simulink model "test_SHState"  (Simulink 6.5)
settings: Solver=VariableStepDiscrete  StartTime=0.0  StopTime=100  RelTol=1e-3
undefined symbols (not defined in the file or in its folder): sigbuilder_block
libraries: xbsIndex_r4 x7, nort_sysgenlib x1
settings Model: Creator=nort  LastModifiedBy=nort

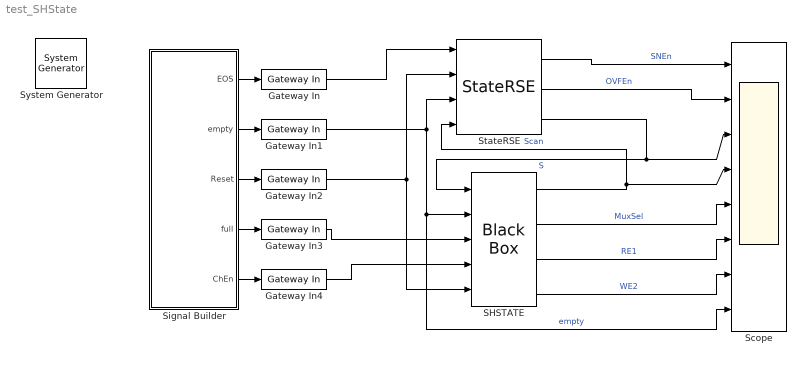
== system test_SHState ==
  " System Generator" : xbsIndex_r4/ System Generator  Tag=genX  SystemSampleTime=-1  xilinxfamily=virtex4  part=xc4vsx35  speed=-10  package=ff668  synthesis_tool=XST  directory=./netlist  testbench=off  simulink_period=1  sysclk_period=10  incr_netlist=off  trim_vbits=Everywhere in SubSystem  dbl_ovrd=According to Block Masks  core_generation=According to Block Masks  run_coregen=off  deprecated_control=off  eval_field=0  block_type=sysgen
      settings: block_version=9.2.01
  Gateway In{,1..3} (4 alike) : xbsIndex_r4/Gateway In  arith_type=Boolean  n_bits=16  bin_pt=14  quantization="Round  (unbiased: +/- Inf)"  overflow=Saturate  period=1  dbl_ovrd=off  timing_constraint=None  locs_specified=off  LOCs={}  block_type=gatewayin
      settings: infoedit="Gateway in block.  Converts inputs of type Simulink integer, double and fixed point to  Xilinx fixed point type.<P><P>Hardware notes:  In hardware these blocks become top level input ports."  block_version=9.2.01
  Gateway In4 : xbsIndex_r4/Gateway In  arith_type=Unsigned  n_bits=3  bin_pt=0  quantization="Round  (unbiased: +/- Inf)"  overflow=Saturate  period=1  dbl_ovrd=off  timing_constraint=None  locs_specified=off  LOCs={}  block_type=gatewayin
      settings: infoedit="Gateway in block.  Converts inputs of type Simulink integer, double and fixed point to  Xilinx fixed point type.<P><P>Hardware notes:  In hardware these blocks become top level input ports."  block_version=9.2.01
  SHSTATE : xbsIndex_r4/Black Box  init_code=SHSTATE_config  sim_method=ISE Simulator  block_type=blackbox2
      settings: infoedit="Incorporates black box HDL and simulation model into a System Generator design.<P><P>You must supply a Black Box with certain information about the HDL component you would like to bring into System Generator. This information is provided through a Matlab function.<P><P>When \"Simulation mode\" is set to \"Inactive\", you will typically want to provide a separate simulation model by using a Simulation Multiplexer.<P>When \"Simulation mode\" is set to \"External co-simulator\", you must include a ModelSim block in the design."  block_version=9.2.01
  Scope : Scope  NumInputPorts=8
      settings: TimeRange=100  YMin=-0.25~-0.25~-0.25~-0.25~-0.1~-0.25~-0.25~-0.25  YMax=1.25~1.25~1.25~1.25~10~1.25~1.25~1.25
  Signal Builder : Subsystem  Tag=STV Subsys  LoadFcn=sigbuilder_block('load');  StartFcn=sigbuilder_block('start');  StopFcn=sigbuilder_block('stop');  ClipboardFcn=sigbuilder_block('clipboard');  mask(Sigbuilder block){}
      mask help: Sigbuilder GUI
      mask init:
      | if ~strcmp(get_param(bdroot(gcbh),'SimulationStatus'),'stopped') tuvar = sigbuilder_block('maskInit'); end
      settings: CopyFcn=sigbuilder_block('copy');  DeleteFcn=sigbuilder_block('delete');  ModelCloseFcn=sigbuilder_block('modelClose');  PreSaveFcn=sigbuilder_block('preSave');  NameChangeFcn=sigbuilder_block('namechange');  OpenFcn=sigbuilder_block('open',[24 64.5 474 399.75 ]);  CloseFcn=sigbuilder_block('close');
      mask Display: plot(0,0,100,100,[10,10,40,40,10],[80,20,20,80,80],[40,10],[50,50], [40,27,10],[65,72,56],[40,25,25,10],[28,28,43,43]);
  StateRSE : nort_sysgenlib/StateRSE  SystemSampleTime=-1
  wires:
  StateRSE/3 -> Scope/3, SHSTATE/1  "S"
  Signal Builder/1(EOS) -> Gateway In/1
  Signal Builder/2(empty) -> Gateway In1/1
  Signal Builder/3(Reset) -> Gateway In2/1
  Signal Builder/4(full) -> Gateway In3/1
  Signal Builder/5(ChEn) -> Gateway In4/1
  StateRSE/1 -> Scope/1  "SNEn"
  StateRSE/2 -> Scope/2  "OVFEn"
  SHSTATE/2 -> Scope/5  "MuxSel"
  SHSTATE/3 -> Scope/6  "RE1"
  SHSTATE/4 -> Scope/7  "WE2"
  Gateway In/1 -> StateRSE/1
  Gateway In1/1 -> StateRSE/3, SHSTATE/2, Scope/8  "empty"
  Gateway In2/1 -> SHSTATE/5, StateRSE/2
  Gateway In3/1 -> SHSTATE/3
  Gateway In4/1 -> SHSTATE/4
  SHSTATE/1 -> Scope/4, StateRSE/4  "Scan"

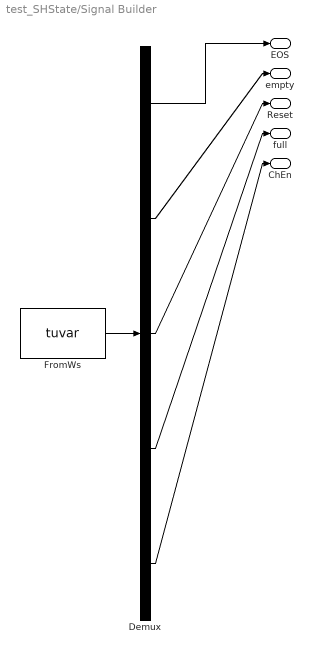
== system test_SHState/Signal Builder ==
  Demux : Demux  Tag=STV Demux  Outputs=5
  FromWs : FromWorkspace  Tag=STV FromWs  VariableName=tuvar  SampleTime=0  SigBuilderData=DataTag1  VnvData=DataTag2
      SigBuilderData=|
      | channels(1).label = 'EOS'
      | channels(1).allXData = {[0 4 6 40 40 41 41 100], [0 4 6 40 40 41 41 100], [0 4 6 40 40 41 41 100], [0 4 6 40 40 41 41 100], [0 4 6 40 40 41 41 100]}
      | channels(1).allYData = {[0 0 0 0 1 1 0 0], [0 0 0 0 1 1 0 0], [0 0 0 0 1 1 0 0], [0 0 0 0 1 1 0 0], [0 0 0 0 1 1 0 0]}
      | channels(2).label = 'empty'
      | channels(2).allXData = {[0 6 6 32 32 37 37 47 47 100], [0 6 6 32 32 37 37 47 47 100], [0 6 6 32 32 37 37 47 47 100], [0 6 6 32 32 37 37 47 47 52 52 100], [0 6 6 32 32 37 37 40 40 41 41 42 42 43 43 100]}
      | channels(2).allYData = {[1 1 0 0 1 1 0 0 1 1], [1 1 0 0 1 1 0 0 1 1], [1 1 0 0 1 1 0 0 1 1], [1 1 0 0 1 1 0 0 1 1 0 0], [1 1 0 0 1 1 0 0 1 1 0 0 1 1 0 0]}
      | channels(3).label = 'Reset'
      | channels(3).allXData = {[0 1 1 2 2 100], [0 1 1 2 2 100], [0 1 1 2 2 100], [0 1 1 2 2 100], [0 1 1 2 2 41 42 100]}
      | channels(3).allYData = {[0 0 1 1 0 0], [0 0 1 1 0 0], [0 0 1 1 0 0], [0 0 1 1 0 0], [0 0 1 1 0 0 0 0]}
      | channels(4).label = 'full'
      | channels(4).allXData = {[0 4 6 43 43 45 45 100], [0 4 6 43 43 45 45 100], [0 4 6 43 43 45 45 100], [0 4 6 43 43 45 45 100], [0 4 6 41 41 48 48 63 63 67 67 100]}
      | channels(4).allYData = {[0 0 0 0 1 1 0 0], [0 0 0 0 1 1 0 0], [0 0 0 0 1 1 0 0], [0 0 0 0 1 1 0 0], [0 0 0 0 1 1 0 0 1 1 0 0]}
      | channels(5).label = 'ChEn'
      | channels(5).allXData = {[0 100], [0 100], [0 100], [0 100], [0 100]}
      | channels(5).allYData = {[7 7], [5 5], [6 6], [4 4], [4 4]}
      | common.afterFinalStr = 'Extrapolate'
      | common.sampleTime = 0
      | dataSet(1).timeRange = [0 100]
      | dataSet(1).name = 'All3'
      | dataSet(2).timeRange = [0 100]
      | dataSet(2).name = 'Ch 0 and 2'
      | dataSet(3).timeRange = [0 100]
      | dataSet(3).name = 'Ch 0 and 1'
      | dataSet(4).timeRange = [0 100]
      | dataSet(4).name = 'Ch 0'
      | dataSet(5).timeRange = [0 100]
      | dataSet(5).name = 'Miss EOS'
  EOS : Outport  Tag=STV Outport
  empty : Outport  Tag=STV Outport  Port=2
  Reset : Outport  Tag=STV Outport  Port=3
  full : Outport  Tag=STV Outport  Port=4
  ChEn : Outport  Tag=STV Outport  Port=5
  wires:
  Demux/1 -> EOS/1
  FromWs/1 -> Demux/1
  Demux/2 -> empty/1
  Demux/3 -> Reset/1
  Demux/4 -> full/1
  Demux/5 -> ChEn/1
